simulink model "A3_LPVMPC_slope_source_isolated"  (R2024b)
settings: Solver=ode4  StartTime=0.0  StopTime=190  FixedStep=0.01  RelTol=1e-3
PreLoadFcn:
  | preloadfcn_v2
model workspace (MAT data in the model file):
  CdA = 0.5
  MPC_idx = [1 2 3 4]
  c_r = 0.015
  db_rt.A = [1 1 1 1 1 1 1 1 1 1 1 1 ... (2000 elements, 5x5x5x4x4)]
  db_rt.B = [1.10696819051e-09 6.56859347141e-11 7.70788358052e-11 4.63456222969e-11 -1.91478442817e-11 3.08062125377e-10 3.17967815903e-10 3.27251111689e-10 3.36091973111e-10 3.44604983367e-10 -2.40695313568e-13 -1.34215112609e-13 ... (1000 elements, 5x5x5x4x2)]
  db_rt.C = [1 1 1 1 1 1 1 1 1 1 1 1 ... (2000 elements, 5x5x5x4x4)]
  db_rt.D = [0 0 0 0 0 0 0 0 0 0 0 0 ... (1000 elements, 5x5x5x4x2)]
  db_rt.E = [2.11033585519e-07 -6.42122832244e-08 -7.53495772598e-08 -4.53058513965e-08 1.871832239e-08 -3.01151562194e-07 -3.10835010863e-07 -3.19910021986e-07 -3.2855251907e-07 -3.36874515032e-07 2.35296065713e-10 1.31204413144e-10 ... (500 elements, 5x5x5x4)]
  db_rt.grid.V = [0.8; 0.9; 1; 1.1; 1.2]
  db_rt.grid.W = [-0.2; -0.1; 0; 0.1; 0.2]
  db_rt.grid.T = [-0.1; -0.05; 0; 0.05; 0.1]
  db_rt.Ts = 0.01
  db_rt.nx = 4
  db_rt.nu = 2
  db_rt.ny = 4
  db_rt.nd = 1
  db_rt.Nv = 5
  db_rt.Nw = 5
  db_rt.Nt = 5
  g = 9.81
  m = 100
  rho = 1.225
undefined symbols (not defined in the file): ff_rt, params, v_ff_nom
libraries: mpclib x1
settings Model: Creator=15754  LastModifiedBy=15754
settings DataIOCC: SaveState=on  LoggingToFile=on  LoggingFileName=ModernTCN_out.mat

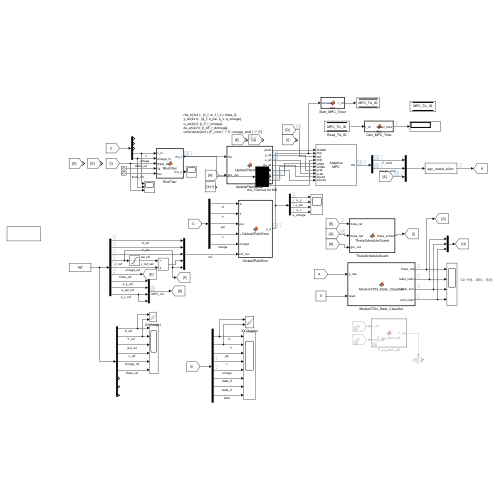
[thumbnail: Simulink's stored preview of the top-level diagram]
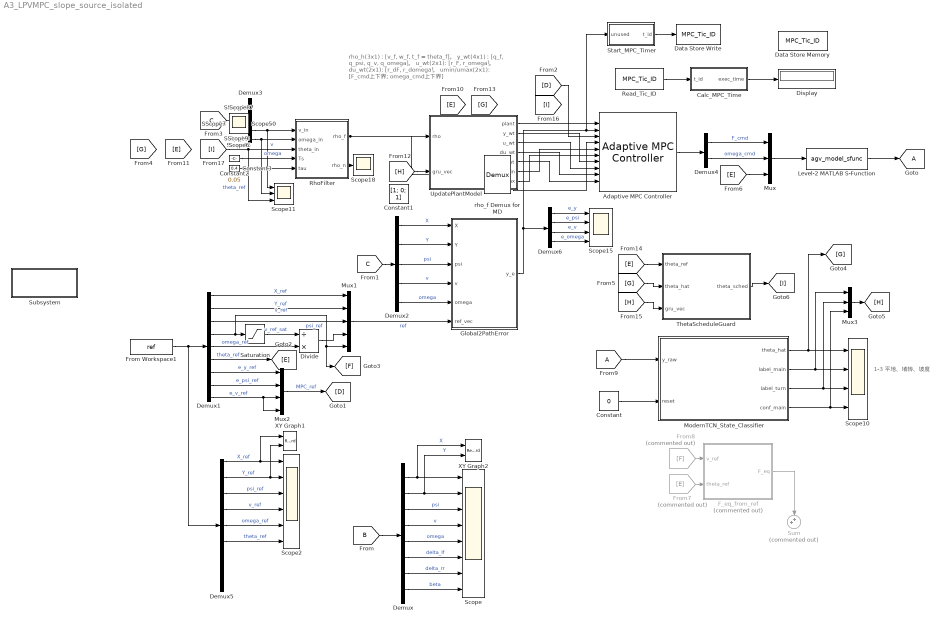
== system A3_LPVMPC_slope_source_isolated ==
  note: rho_h(3x1)：[v_f, w_f, t_f = theta_f]。
      | y_wt(4x1)：[q_f, q_psi, q_v, q_omega]。
      | u_wt(2x1): [r_F, r_omega]。
      | du_wt(2x1): [r_dF, r_domega]。
      | umin/umax(2x1): [F_cmd上下界; omega_cmd上下界]
  note: 1-3 平地、堵转、坡度
  Adaptive MPC Controller : mpclib/Adaptive MPC Controller  SCDEnableBlockLinearizationSpecification=on  mpcobj=ctrl.mpcobj  enable_value=0  updateMPCinCallerWorkspace=on  md_inport=on  mv_inport=off  uref_inport=off  return_cost=off  return_mvseq=off  return_qpstatus=off  return_xseq=off  return_state=off  return_ovseq=off  state_inport=off  isltv_plant=off  umin_inport=on  umax_inport=on  ymin_inport=off  ymax_inport=off  cc_inport=off  ywt_inport=on  uwt_inport=on  duwt_inport=on  rhoeps_inport=on  pm_inport=off  MaximumP=10  HorizonChoice=FixedHorizon  BlockDataType=double  SampleTimeInherited=off  switch_inport=off
  Calc_MPC_Time : MATLAB Function  TreatAsAtomicUnit=on
  Constant : Constant  Value=0  SampleTime=params.Ts
  Constant1 : Constant  Value=[1; 0; 1]  SampleTime=0.01
  Constant2 : Constant  Value=0.05  SampleTime=params.Ts
  Constant3 : Constant  Value=0.4  SampleTime=params.Ts
  Data Store Memory : DataStoreMemory  DataStoreName=MPC_Tic_ID  WriteAfterWriteMsg=warning  ShowAdditionalParam=off  OutDataTypeStr=uint64  DataLoggingName=solve_time_ms
      settings: DataLoggingNameMode=Custom
  Data Store Write : DataStoreWrite  DataStoreName=MPC_Tic_ID  IndexOptions=Index vector (dialog)  Indices=1  OutputSizes=1
  Demux : Demux  Outputs=8
  Demux1 : Demux  Outputs=9
  Demux2 : Demux  Outputs=5
  Demux3 : Demux  Outputs=5
  Demux4 : Demux  Outputs=2
  Demux5 : Demux  Outputs=9
  Demux6 : Demux
  Display : Display
  Divide : Product  Inputs=/*
  F_eq_from_ref : MATLAB Function  Commented=on  TreatAsAtomicUnit=on
  From Workspace1 : FromWorkspace  VariableName=ref  SampleTime=0.05
  From7 : From  Commented=on  GotoTag=E
  From8 : From  Commented=on  GotoTag=F
  From9 : From  TagVisibility=global
  Global2PathError : MATLAB Function  TreatAsAtomicUnit=on  SystemSampleTime=params.Ts
  Goto : Goto  TagVisibility=global
  Level-2 MATLAB S-Function : M-S-Function  FunctionName=agv_model_sfunc  Parameters=parameters
  ModernTCN_State_Classifier : MATLAB Function  TreatAsAtomicUnit=on
  Mux : Mux  Inputs=3
  Mux1 : Mux  Inputs=5
  Mux2 : Mux
  Mux3 : Mux  Inputs=3
  Read_Tic_ID : DataStoreRead  DataStoreName=MPC_Tic_ID  IndexOptions=Index vector (dialog)  Indices=1  OutputSizes=1
  RhoFilter : MATLAB Function  TreatAsAtomicUnit=on  SystemSampleTime=0.05
  Saturation : Saturate  UpperLimit=Inf  LowerLimit=1e-3
  Scope : Scope  NumInputPorts=8
  Scope10 : Scope  NumInputPorts=4
  Scope11 : Scope  NumInputPorts=3
  Scope15 : Scope  NumInputPorts=4
  Scope{1,3..9,12..14,16..22} (18 alike) : Scope
  Scope2 : Scope  NumInputPorts=6
  Start_MPC_Timer : MATLAB Function  TreatAsAtomicUnit=on
  Subsystem : Subsystem
  Sum : Sum  Commented=on  Inputs=++|
  ThetaScheduleGuard : MATLAB Function  TreatAsAtomicUnit=on
  UpdatePlantModel : MATLAB Function  TreatAsAtomicUnit=on
  XY Graph1 : Record  FileSettingsInternal="{\"entries\":[{\"content\":{\"excelSettings\":{\"content\":{},\"type\":\"Streamout.ExcelSettings\"}},\"type\":\"Streamout.FileSettingStorage\",\"uuid\":\"\"}],\"packageUris\":[\"http:\\/\\/schema.mathworks.com\\/mf0\\/streamout_blocks\\/R2020a\"],\"version\":\"1.0\"}"  Layout=[1 1]  SignalsInternal="{\"entries\":[{\"content\":{\"signals\":[{\"content\":{\"blockPath\":[],\"dimensions\":[1],\"domain\":\"\",\"lineColor\":\"#a2142f\",\"plots\":[ 1 ],\"port\":1,\"signalID\":1,\"signalName\":\"X_ref\"},\"type\":\"RecordBlkView.Signal\",\"uuid\":\"\"},{\"content\":{\"blockPath\":[],\"dimensions\":[1],\"domain\":\"\",\"lineColor\":\"#139fff\",\"plots\":[ 1 ],\"port\":2,\"signalID\":2,\"signalName\":\"Y_ref\"},\"type\":\"RecordBlkView.Signal\",\"uuid\":\"\"}]},\"type\":\"RecordBlkView.InputSignals\",\"uuid\":\"\"}],\"packageUris\":[\"http:\\/\\/schema.mathworks.com\\/mf0\\/streamout_blocks\\/R2020a\"],\"version\":\"1.0\"}"  VisualizationBindings="{\"xyplotplugin\":{\"info\":[{\"series\":[{\"bindingParametersList\":[{\"parameter\":\"X-Axis\",\"signalID\":1,\"signalName\":\"X_ref\"},{\"parameter\":\"Y-Axis\",\"signalID\":2,\"signalName\":\"Y_ref\"}],\"seriesID\":0}],\"subplotID\":1}]}}"  CompatibilityTag=XY
  XY Graph2 : Record  FileSettingsInternal="{\"entries\":[{\"content\":{\"excelSettings\":{\"content\":{},\"type\":\"Streamout.ExcelSettings\"}},\"type\":\"Streamout.FileSettingStorage\",\"uuid\":\"\"}],\"packageUris\":[\"http:\\/\\/schema.mathworks.com\\/mf0\\/streamout_blocks\\/R2020a\"],\"version\":\"1.0\"}"  Layout=[1 1]  SignalsInternal="{\"entries\":[{\"content\":{\"signals\":[{\"content\":{\"blockPath\":[],\"dimensions\":[1],\"domain\":\"\",\"lineColor\":\"#a2142f\",\"plots\":[ 1 ],\"port\":1,\"signalID\":1,\"signalName\":\"X\"},\"type\":\"RecordBlkView.Signal\",\"uuid\":\"\"},{\"content\":{\"blockPath\":[],\"dimensions\":[1],\"domain\":\"\",\"lineColor\":\"#139fff\",\"plots\":[ 1 ],\"port\":2,\"signalID\":2,\"signalName\":\"Y\"},\"type\":\"RecordBlkView.Signal\",\"uuid\":\"\"}]},\"type\":\"RecordBlkView.InputSignals\",\"uuid\":\"\"}],\"packageUris\":[\"http:\\/\\/schema.mathworks.com\\/mf0\\/streamout_blocks\\/R2020a\"],\"version\":\"1.0\"}"  VisualizationBindings="{\"xyplotplugin\":{\"info\":[{\"series\":[{\"bindingParametersList\":[{\"parameter\":\"X-Axis\",\"signalID\":1,\"signalName\":\"X\"},{\"parameter\":\"Y-Axis\",\"signalID\":2,\"signalName\":\"Y\"}],\"seriesID\":0}],\"subplotID\":1}]}}"  CompatibilityTag=XY
  rho_f Demux for MD : Demux  Outputs=3
  wires:
  Level-2 MATLAB S-Function/1 -> Goto/1
  [B] -> Demux/1
  Demux/1 -> XY Graph2/1, Scope/1  "X"
  Demux/2 -> XY Graph2/2, Scope/2  "Y"
  Demux/3 -> Scope/3  "psi"
  Demux/4 -> Scope/4  "v"
  Demux/5 -> Scope/5  "omega"
  Demux/6 -> Scope/6  "delta_lf"
  Demux/7 -> Scope/7  "delta_rr"
  Demux/8 -> Scope/8  "beta"
  Demux1/4 -> [F], Mux1/5, Saturation/1  "v_ref"
  Saturation/1 -> Divide/1  "v_ref_sat"
  Demux1/5 -> Divide/2  "omega_ref"
  Demux1/1 -> Mux1/1  "X_ref"
  Demux1/2 -> Mux1/2  "Y_ref"
  Demux1/3 -> Mux1/3  "psi_ref"
  Divide/1 -> Mux1/4
  Mux1/1 -> Global2PathError/6(ref_vec)  "ref"
  [C] -> Demux2/1
  Demux2/3 -> Global2PathError/3(psi)  "psi"
  Demux2/4 -> Global2PathError/4(v)  "v"
  Demux2/5 -> Global2PathError/5(omega)  "omega"
  Demux2/2 -> Global2PathError/2(Y)  "Y"
  Demux2/1 -> Global2PathError/1(X)  "X"
  Demux1/8 -> Mux2/2  "e_psi_ref"
  Demux1/7 -> Mux2/1  "e_y_ref"
  Demux1/9 -> Mux2/4, Mux2/3  "e_v_ref"
  Mux2/1 -> [D]  "MPC_ref"
  [D] -> Adaptive MPC Controller/3
  [C] -> Demux3/1
  Demux3/4 -> Scope11/1, RhoFilter/1(v_in)  "v"
  Demux3/5 -> Scope11/2, RhoFilter/2(omega_in)  "omega"
  Demux1/6 -> [E]  "theta_ref"
  [I] -> Scope11/3, RhoFilter/3(theta_in)  "theta_ref"
  Constant2/1 -> RhoFilter/4(Ts)
  Constant3/1 -> RhoFilter/5(tau)
  UpdatePlantModel/1(plant) -> Adaptive MPC Controller/1
  RhoFilter/1(rho_f) -> UpdatePlantModel/1(rho), rho_f Demux for MD/1
  Demux5/1 -> XY Graph1/1, Scope2/1  "X_ref"
  Demux5/2 -> XY Graph1/2, Scope2/2  "Y_ref"
  Demux5/3 -> Scope2/3  "psi_ref"
  Demux5/4 -> Scope2/4  "v_ref"
  Demux5/5 -> Scope2/5  "omega_ref"
  Demux5/6 -> Scope2/6  "theta_ref"
  UpdatePlantModel/6(umin) -> Adaptive MPC Controller/5
  UpdatePlantModel/7(umax) -> Adaptive MPC Controller/6
  UpdatePlantModel/2(y_wt) -> Adaptive MPC Controller/7
  UpdatePlantModel/3(u_wt) -> Adaptive MPC Controller/8
  UpdatePlantModel/4(du_wt) -> Adaptive MPC Controller/9
  UpdatePlantModel/5(ecr_wt) -> Adaptive MPC Controller/10
  Global2PathError/1(y_e) -> Demux6/1, Start_MPC_Timer/1(unused), Adaptive MPC Controller/2
  Mux/1 -> Level-2 MATLAB S-Function/1
  Adaptive MPC Controller/1 -> Demux4/1
  [E] -> Mux/3
  Demux4/2 -> Mux/2  "omega_cmd"
  F_eq_from_ref/1(F_eq) -> Sum/1
  From8/1 -> F_eq_from_ref/1(v_ref)
  From7/1 -> F_eq_from_ref/2(theta_ref)
  Demux4/1 -> Mux/1  "F_cmd"
  From9/1 -> ModernTCN_State_Classifier/1(y_raw)
  ModernTCN_State_Classifier/4(conf_main) -> Mux3/3, Scope10/4
  ModernTCN_State_Classifier/2(label_main) -> Mux3/1, Scope10/2
  Constant/1 -> ModernTCN_State_Classifier/2(reset)
  ModernTCN_State_Classifier/3(label_turn) -> Mux3/2, Scope10/3
  ModernTCN_State_Classifier/1(theta_hat) -> [G], Scope10/1
  From Workspace1/1 -> Demux5/1, Demux1/1
  Demux6/1 -> Scope15/1  "e_y"
  Demux6/2 -> Scope15/2  "e_psi"
  Demux6/3 -> Scope15/3  "e_v"
  Demux6/4 -> Scope15/4  "e_omega"
  RhoFilter/2(rho_n) -> Scope18/1
  Mux3/1 -> [H]
  [H] -> UpdatePlantModel/2(gru_vec)
  Start_MPC_Timer/1(t_id) -> Data Store Write/1
  Read_Tic_ID/1 -> Calc_MPC_Time/1(t_id)
  Calc_MPC_Time/1(exec_time) -> Display/1
  [G] -> ThetaScheduleGuard/2(theta_hat)
  [E] -> ThetaScheduleGuard/1(theta_ref)
  [H] -> ThetaScheduleGuard/3(gru_vec)
  ThetaScheduleGuard/1(theta_sched) -> [I]
  rho_f Demux for MD/3 -> Adaptive MPC Controller/4

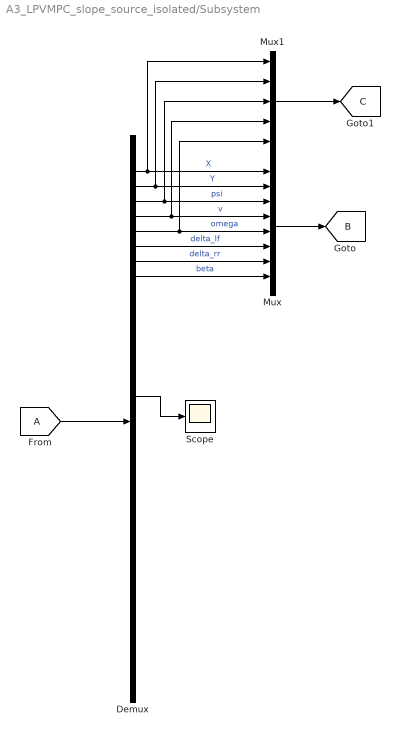
== system A3_LPVMPC_slope_source_isolated/Subsystem ==
  Demux : Demux  Outputs=34
  From : From  TagVisibility=global
  Mux : Mux  Inputs=8
  Mux1 : Mux  Inputs=5
  Scope : Scope
  tag scope: B=global, C=global
  wires:
  From/1 -> Demux/1
  Demux/1 -> Mux/1, Mux1/1  "X"
  Demux/2 -> Mux/2, Mux1/2  "Y"
  Demux/3 -> Mux/3, Mux1/3  "psi"
  Demux/4 -> Mux/4, Mux1/4  "v"
  Demux/5 -> Mux/5, Mux1/5  "omega"
  Demux/6 -> Mux/6  "delta_lf"
  Demux/7 -> Mux/7  "delta_rr"
  Demux/8 -> Mux/8  "beta"
  Mux/1 -> [B]
  Mux1/1 -> [C]
  Demux/16 -> Scope/1

== matlab function A3_LPVMPC_slope_source_isolated/Start_MPC_Timer ==
  data: unused input; t_id output
function t_id = fcn(~)
%#codegen
% 声明tic为 extrinsic 函数，避免代码生成报错
coder.extrinsic('tic');
t_id = uint64(0);
t_id = tic; % 启动计时器，获取句柄

== matlab function A3_LPVMPC_slope_source_isolated/ThetaScheduleGuard ==
  data: theta_ref input double size=[1 1]; theta_sched output double size=[1 1]; theta_hat input double size=[1 1]; gru_vec input double size=[3 1]; a3_theta_mode parameter double size=[1 1]
function theta_sched = ThetaScheduleGuard(theta_ref, theta_hat, gru_vec, a3_theta_mode)
%#codegen
% A3 frozen mode: 1=ZS, 2=causal IMU, 3=Oracle. gru_vec is intentionally unused.
mode = round(double(a3_theta_mode(1)));
theta_lim = deg2rad(12.0);
theta_ref_scalar = double(theta_ref(1));
theta_hat_scalar = double(theta_hat(1));
theta_sched = 0.0;
if mode == 1
    theta_sched = 0.0;
elseif mode == 2
    theta_sched = min(theta_lim, max(-theta_lim, theta_hat_scalar));
elseif mode == 3
    theta_sched = min(theta_lim, max(-theta_lim, theta_ref_scalar));
else
    theta_sched = 0.0;
end
end

== matlab function A3_LPVMPC_slope_source_isolated/RhoFilter ==
  data: v_in input; rho_f output; omega_in input; theta_in input; Ts input; tau input; rho_n output
function [rho_f, rho_n] = RhoFilter(v_in, omega_in, theta_in, Ts, tau)
% 一阶离散滤波
persistent v_f_prev w_f_prev t_f_prev
if isempty(v_f_prev), v_f_prev = 0; end
if isempty(w_f_prev), w_f_prev = 0; end
if isempty(t_f_prev), t_f_prev = 0; end

a = Ts / max(tau + Ts, 1e-6);

v_f = (1 - a)*v_f_prev + a*max(v_in, 0);   % 速度不取负·
w_f = (1 - a)*w_f_prev + a*omega_in;       % 保留符号
t_f = (1 - a)*t_f_prev + a*theta_in;       % 保留符号

v_f_prev = v_f; w_f_prev = w_f; t_f_prev = t_f;

rho_f = [v_f; w_f; t_f];

% 可选归一化（仅用于监控/调试，不参与UpdatePlantModel）
Vmax = 2.0; Wmax = 0.8; Tmax = deg2rad(10);
rho_n = [min(v_f/Vmax,1); min(abs(w_f)/Wmax,1); min(abs(t_f)/Tmax,1)];
end

== matlab function A3_LPVMPC_slope_source_isolated/Global2PathError ==
  data: X input; y_e output; Y input; psi input; v input; omega input; ref_vec input
% 误差计算模块
function y_e = Global2PathError(X, Y, psi, v, omega, ref_vec)
% ref_vec = [X_ref; Y_ref; psi_ref; kappa_ref; v_ref]
% 输出: y_e = [e_y; e_psi; e_v; e_omega; e_s]

%#codegen
% 1) 解包参考
Xr = ref_vec(1);
Yr = ref_vec(2);
psir = ref_vec(3);
kappa = ref_vec(4);
v_ref = ref_vec(5);

% 2) 横向误差：沿参考法向量投影（带符号）
ex = X - Xr; 
ey = Y - Yr;
e_y = -sin(psir)*ex + cos(psir)*ey;

% 3) 航向、速度、角速度误差
e_psi   = wrapToPi(psi - psir);
e_v     = v - v_ref;
omega_ff= v_ref * kappa;           % 曲率前馈
e_omega = omega - omega_ff;

% 4) 进度误差（可选，如未使用可置 0）
e_s = 0;

y_e = [e_y; e_psi; e_v; e_omega];
end

== matlab function A3_LPVMPC_slope_source_isolated/UpdatePlantModel ==
  data: rho input; gru_vec input; plant output Bus: MPCPlantBus; db_rt parameter; MPC_idx parameter double size=[1 4]; ff_rt parameter; v_ff_nom parameter; y_wt output; u_wt output; du_wt output; ecr_wt output; umin output; umax output
function [plant, y_wt, u_wt, du_wt, ecr_wt, umin, umax] = UpdatePlantModel(rho, gru_vec, db_rt, MPC_idx, ff_rt, v_ff_nom)
%#codegen
% gru_vec = [label_main; label_turn; conf_main]

gv = [1; 0; 1]; % 默认: flat / straight / high confidence
if ~isempty(gru_vec)
g = double(gru_vec(:));
n = min(3, numel(g));
gv(1:n) = g(1:n);
end

[plant, y_wt, u_wt, du_wt, ecr_wt, umin, umax] = UpdatePlantModel_gru( ...
rho, db_rt, MPC_idx, ff_rt, v_ff_nom, gv);
end

== matlab function A3_LPVMPC_slope_source_isolated/F_eq_from_ref ==
  data: v_ref input; F_eq output; theta_ref input; m parameter double; g parameter double; c_r parameter double; rho parameter double; CdA parameter double
function F_eq = F_eq_from_ref(v_ref, theta_ref, m, g, c_r, rho, CdA)
%#codegen
% v_ref, theta_ref: 输入端口
% m,g,c_r,rho,CdA  : 本块的 Parameter（标量 double）
v = max(v_ref, 0);
F_roll = c_r * m * g * cos(theta_ref);
F_aero = 0.5 * rho * CdA .* (v.^2);
F_eq = F_roll + F_aero;

% 保持“前馈不含 m·g·sinθ”，以免与 MD 通道重复补偿。

== matlab function A3_LPVMPC_slope_source_isolated/Calc_MPC_Time ==
  data: t_id input; exec_time output
function exec_time = fcn(t_id)
%#codegen
% 声明toc为 extrinsic 函数
coder.extrinsic('toc');
exec_time = 0;
exec_time = toc(t_id); % 计算耗时，单位：秒

== matlab function A3_LPVMPC_slope_source_isolated/ModernTCN_State_Classifier ==
  data theta_hat settings: description=坡度角估计 (rad)
  data label_main settings: description=主分类 [1,2,3,4]
  data label_turn settings: description=转弯状态 [-1, 0, 1]
  data conf_main settings: description=主分类置信度 [0, 1]
  data: y_raw input double size=[34 1]; theta_hat output double size=[1 1]; reset input double size=[1 1]; label_main output double size=[1 1]; label_turn output double size=[1 1]; conf_main output double size=[1 1]
function [theta_hat, label_main, label_turn, conf_main] = ModernTCN_State_Classifier(y_raw, reset)
%#codegen
coder.extrinsic('A3_Causal_IMU_Theta_sim');
theta_hat = 0.0;
theta_hat = A3_Causal_IMU_Theta_sim(y_raw, reset);
label_main = 1.0;
label_turn = 0.0;
conf_main = 1.0;
end
